simulink model "enabledSubsystem_example"  (R2017a)
settings: Solver=VariableStepAuto  StartTime=0.0  StopTime=10.0  RelTol=1e-3
settings Model: Creator=edward  LastModifiedBy=edward

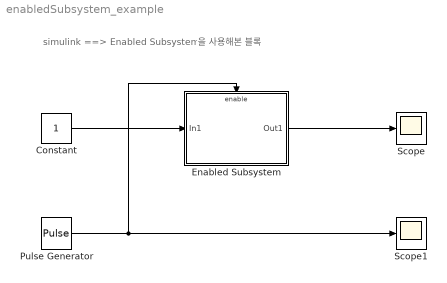
== system enabledSubsystem_example ==
  note: simulink ==> Enabled Subsystem을 사용해본 블록
  Constant : Constant
  "Enabled Subsystem " : Subsystem
  Pulse Generator : DiscretePulseGenerator  PulseType=Time based  PulseWidth=50
  Scope : Scope
  Scope1 : Scope
  wires:
  Pulse Generator/1 -> "Enabled Subsystem "/Enable, Scope1/1
  Constant/1 -> "Enabled Subsystem "/1(In1)
  "Enabled Subsystem "/1(Out1) -> Scope/1

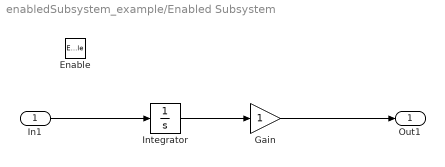
== system enabledSubsystem_example/Enabled Subsystem  ==
  In1 : Inport
  Enable : EnablePort
  Gain : Gain
  Integrator : Integrator
  Out1 : Outport
  wires:
  In1/1 -> Integrator/1
  Integrator/1 -> Gain/1
  Gain/1 -> Out1/1
